simulink model "bfsk"  (Simulink 6.4)
settings: Solver=FixedStepDiscrete  SolverMode=SingleTasking  StartTime=0.0  StopTime=20  RelTol=1e-3
undefined symbols (not defined in the file or in its folder): Fs, get
libraries: commsink2 x3, commdigbbndfm2 x2, commchan3 x1, commdigbbndcpm2 x1, commrandsrc2 x1, dspsnks4 x1
settings Model: Creator=ALEX  LastModifiedBy=student
settings OptimizationCC: InitFltsAndDblsToZero=off
settings DebuggingCC: SignalResolutionControl=UseLocalSettings  MultiTaskDSMMsg=error  MultiTaskCondExecSysMsg=error
settings GRTTargetCC: TargetFcnLib=ansi_tfl_table_tmw.mat

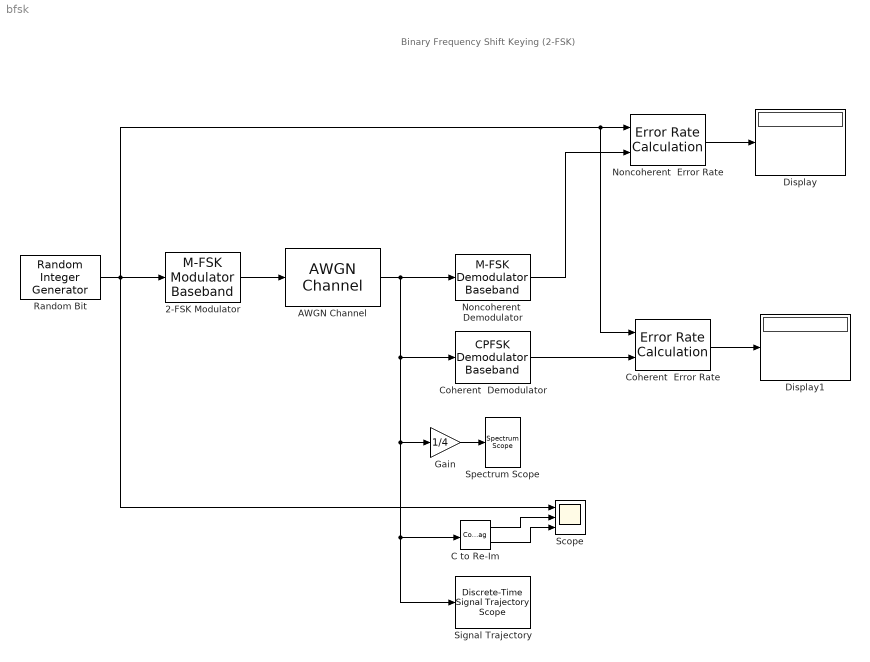
== system bfsk ==
  note: Binary Frequency Shift Keying (2-FSK)
  2-FSK Modulator : commdigbbndfm2/M-FSK Modulator Baseband  M=2  InType=Bit  Enc=Binary  freqSep=1  phaseType=Continuous  numSamp=16  outDataType=double
  AWGN Channel : commchan3/AWGN Channel  SystemSampleTime=-1  seed=67  noiseMode="Signal to noise ratio  (Es/No)"  EbNodB=3  EsNodB=100  SNRdB=6  bitsPerSym=1  Ps=1  Tsym=1  variance=16
  C to Re-Im : ComplexToRealImag
  Coherent  Demodulator : commdigbbndcpm2/CPFSK Demodulator Baseband  SystemSampleTime=-1  Mnum=2  outputType=Bit  mappingType=Binary  modIdx=1  phaseOffset=0  samplesPerSymbol=16  traceBack=4  outDtype=boolean
  Coherent  Error Rate : commsink2/Error Rate Calculation  N=5  st_delay=0  cp_mode=Entire frame  subframe=[]  PMode=Port  WsName=ErrorVec  RsMode2=off  stop=off  numErr=1000  maxBits=100000
  Display : Display
  Display1 : Display
  Gain : Gain  Gain=1/4  ParameterDataType=fixdt(1, 16)  OutDataType=fixdt(1, 16)
  Noncoherent  Demodulator : commdigbbndfm2/M-FSK Demodulator Baseband  M=2  OutType=Bit  Dec=Binary  freqSep=1  numSamp=16  outDataType=boolean
  Noncoherent  Error Rate : commsink2/Error Rate Calculation  N=1  st_delay=0  cp_mode=Entire frame  subframe=[]  PMode=Port  WsName=ErrorVec  RsMode2=off  stop=off  numErr=1000  maxBits=100000
  Random Bit : commrandsrc2/Random Integer Generator  SystemSampleTime=-1  mul=2  seed=57  Ts=1  frameBased=off  sampPerFrame=8  orient=off  outDataType=boolean
  Scope : Scope  NumInputPorts=3
      settings: YMin=0~-3~-3  YMax=1.2~3~3
  Signal Trajectory : commsink2/Discrete-Time Signal Trajectory Scope  Tag=SignalTrajectory  SystemSampleTime=-1  sampPerSymb=64  offsetEye=0  numTraces=1  numNewFrames=1  LineStyles=-  LineColors=b  fading=on  render=on  AxisGrid=on  xMin=-2  xMax=2  yMin=-2  yMax=2  inphaseLabel=In-phase Amplitude  quadratureLabel=Quadrature Amplitude  openScopeAtSimStart=off  FrameNumber=off  FigPos=get(0,'defaultfigureposition');  figTitle=Signal Trajectory  numLinesMax=8  block_type_=xy
  Spectrum Scope : dspsnks4/Spectrum Scope  DialogController=dspdialog.SpectrumScope  DialogControllerArgs=DataTag0  SystemSampleTime=-1  ScopeProperties=on  Domain=Frequency  HorizSpan=1  UseBuffer=on  BufferSize=2048  Overlap=0  inpFftLenInherit=off  FFTlength=128  numAvg=40  DisplayProperties=off  AxisGrid=on  Memory=off  FrameNumber=on  AxisLegend=off  AxisZoom=off  OpenScopeAtSimStart=off  OpenScopeImmediately=off  FigPos=get(0,'defaultfigureposition')  AxisProperties=off  XUnits=Hertz  XRange=[-Fs/2...Fs/2]  InheritXIncr=on  XIncr=1.0  XLabel=Samples  YUnits=dB  YLabel=Magnitude-squared, dB  LineProperties=off  LineColors=[1 0 0]  wintypeSpecScope=Hamming  RsSpecScope=50  betaSpecScope=5  winsampSpecScope=Periodic
      settings: YMin=-10  YMax=10
  wires:
  Noncoherent  Error Rate/1 -> Display/1
  AWGN Channel/1 -> Noncoherent  Demodulator/1, Coherent  Demodulator/1, Gain/1, Signal Trajectory/1, C to Re-Im/1
  Random Bit/1 -> 2-FSK Modulator/1, Noncoherent  Error Rate/1, Coherent  Error Rate/1, Scope/1
  Coherent  Error Rate/1 -> Display1/1
  Noncoherent  Demodulator/1 -> Noncoherent  Error Rate/2
  Coherent  Demodulator/1 -> Coherent  Error Rate/2
  2-FSK Modulator/1 -> AWGN Channel/1
  Gain/1 -> Spectrum Scope/1
  C to Re-Im/1 -> Scope/2
  C to Re-Im/2 -> Scope/3
